simulink model "InjCrv_MI1Cor"  (R2016b)
settings: configuration reference "CodeGenConfigSet" (kept outside this file)
values from neighbouring files (symbols this model uses):
  InjCrv_facMI1APSSOECor_CUR = Calibration.Parameter    [init_InjCrv_MI1Cor.m]
  InjCrv_facMI1APSSOECor_CURX = Calibration.Parameter    [init_InjCrv_MI1Cor.m]
  InjCrv_facMI1ATSSOECor_CUR = Calibration.Parameter    [init_InjCrv_MI1Cor.m]
  InjCrv_facMI1ATSSOECor_CURX = Calibration.Parameter    [init_InjCrv_MI1Cor.m]
  InjCrv_facMI1ETSSOECor_CUR = Calibration.Parameter    [init_InjCrv_MI1Cor.m]
  InjCrv_facMI1ETSSOECor_CURX = Calibration.Parameter    [init_InjCrv_MI1Cor.m]
  InjCrv_phiMI1APSCor1EOM_MAP = Calibration.Parameter    [init_InjCrv_MI1Cor.m]
  InjCrv_phiMI1APSCor1EOM_MAPX = Calibration.Parameter    [init_InjCrv_MI1Cor.m]
  InjCrv_phiMI1APSCor1EOM_MAPY = Calibration.Parameter    [init_InjCrv_MI1Cor.m]
  InjCrv_phiMI1ATSCor1EOM_MAP = Calibration.Parameter    [init_InjCrv_MI1Cor.m]
  InjCrv_phiMI1ATSCor1EOM_MAPX = Calibration.Parameter    [init_InjCrv_MI1Cor.m]
  InjCrv_phiMI1ATSCor1EOM_MAPY = Calibration.Parameter    [init_InjCrv_MI1Cor.m]
  InjCrv_phiMI1ETSCor1EOM_MAP = Calibration.Parameter    [init_InjCrv_MI1Cor.m]
  InjCrv_phiMI1ETSCor1EOM_MAPX = Calibration.Parameter    [init_InjCrv_MI1Cor.m]
  InjCrv_phiMI1ETSCor1EOM_MAPY = Calibration.Parameter    [init_InjCrv_MI1Cor.m]
settings Model: Creator=Administrator  LastModifiedBy=wangrui
settings ConfigSetRef: SourceLocation=Base Workspace

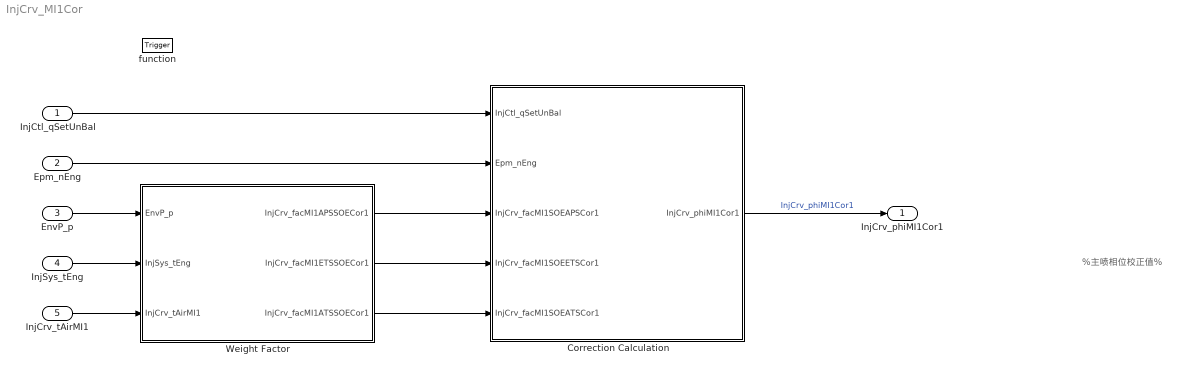
== system InjCrv_MI1Cor ==
  note: %主喷相位校正值%
  InjCtl_qSetUnBal : Inport  Tag=mg/hub  Description=Current injection quantity  OutMin=-319  OutMax=319  OutDataTypeStr=FuelMass_mg_hub
  Epm_nEng : Inport  Tag=rpm  Description=Engine speed  Port=2  OutMin=0  OutMax=6000  OutDataTypeStr=EngSpeed_rpm
  EnvP_p : Inport  Tag=kPa  Description=Barometric pressure  Port=3  OutMin=0  OutMax=3276  OutDataTypeStr=AirPressure_kPa
  InjSys_tEng : Inport  Tag=deg  Description=Engine temperature selected for the injection system  Port=4  OutMin=-1000  OutMax=1000  OutDataTypeStr=Temp_deg
  InjCrv_tAirMI1 : Inport  Tag=deg  Description=Chosen temperature from the temperature field on the induction system  Port=5  OutMin=-50  OutMax=150  OutDataTypeStr=Temp_deg
  function : TriggerPort  TriggerType=function-call  VariantControl=Variant
  Correction Calculation : Subsystem
  Weight Factor : Subsystem
  InjCrv_phiMI1Cor1 : Outport  Tag=CA  Description=Start of energizing correction for MI1  OutMin=-40  OutMax=40  OutDataTypeStr=Angle_CA
  wires:
  EnvP_p/1 -> Weight Factor/1(EnvP_p)
  InjSys_tEng/1 -> Weight Factor/2(InjSys_tEng)
  InjCrv_tAirMI1/1 -> Weight Factor/3(InjCrv_tAirMI1)
  InjCtl_qSetUnBal/1 -> Correction Calculation/1(InjCtl_qSetUnBal)
  Epm_nEng/1 -> Correction Calculation/2(Epm_nEng)
  Weight Factor/1(InjCrv_facMI1APSSOECor1) -> Correction Calculation/3(InjCrv_facMI1SOEAPSCor1)
  Weight Factor/2(InjCrv_facMI1ETSSOECor1) -> Correction Calculation/4(InjCrv_facMI1SOEETSCor1)
  Weight Factor/3(InjCrv_facMI1ATSSOECor1) -> Correction Calculation/5(InjCrv_facMI1SOEATSCor1)
  Correction Calculation/1(InjCrv_phiMI1Cor1) -> InjCrv_phiMI1Cor1/1  "InjCrv_phiMI1Cor1"

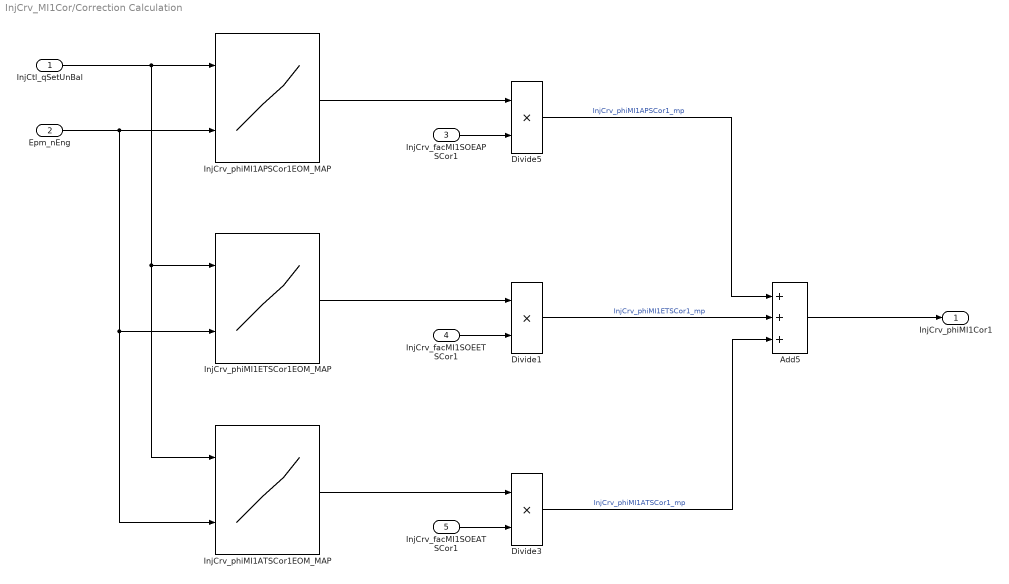
== system InjCrv_MI1Cor/Correction Calculation ==
  InjCtl_qSetUnBal : Inport
  Epm_nEng : Inport  Port=2
  InjCrv_facMI1SOEAPSCor1 : Inport  Port=3
  InjCrv_facMI1SOEETSCor1 : Inport  Port=4
  InjCrv_facMI1SOEATSCor1 : Inport  Port=5
  Add5 : Sum  Inputs=+++  SaturateOnIntegerOverflow=on  InputSameDT=on
  Divide1 : Product  Inputs=**  OutDataTypeStr=Inherit: Inherit via back propagation
  Divide3 : Product  Inputs=**  OutDataTypeStr=Inherit: Inherit via back propagation
  Divide5 : Product  Inputs=**  OutDataTypeStr=Inherit: Inherit via back propagation
  InjCrv_phiMI1APSCor1EOM_MAP : Lookup_n-D  BreakpointsForDimension1=InjCrv_phiMI1APSCor1EOM_MAPY  BreakpointsForDimension2=InjCrv_phiMI1APSCor1EOM_MAPX  IndexSearchMethod=Linear search  BeginIndexSearchUsingPreviousIndexResult=on  Table=InjCrv_phiMI1APSCor1EOM_MAP  ExtrapMethod=Clip  UseLastTableValue=on  InternalRulePriority=Speed  OutDataTypeStr=Inherit: Inherit via back propagation  SaturateOnIntegerOverflow=on
  InjCrv_phiMI1ATSCor1EOM_MAP : Lookup_n-D  BreakpointsForDimension1=InjCrv_phiMI1ATSCor1EOM_MAPY  BreakpointsForDimension2=InjCrv_phiMI1ATSCor1EOM_MAPX  IndexSearchMethod=Linear search  BeginIndexSearchUsingPreviousIndexResult=on  Table=InjCrv_phiMI1ATSCor1EOM_MAP  ExtrapMethod=Clip  UseLastTableValue=on  InternalRulePriority=Speed  OutDataTypeStr=Inherit: Inherit via back propagation  SaturateOnIntegerOverflow=on
  InjCrv_phiMI1ETSCor1EOM_MAP : Lookup_n-D  BreakpointsForDimension1=InjCrv_phiMI1ETSCor1EOM_MAPY  BreakpointsForDimension2=InjCrv_phiMI1ETSCor1EOM_MAPX  IndexSearchMethod=Linear search  BeginIndexSearchUsingPreviousIndexResult=on  Table=InjCrv_phiMI1ETSCor1EOM_MAP  ExtrapMethod=Clip  UseLastTableValue=on  InternalRulePriority=Speed  OutDataTypeStr=Inherit: Inherit via back propagation  SaturateOnIntegerOverflow=on
  InjCrv_phiMI1Cor1 : Outport
  wires:
  InjCrv_phiMI1APSCor1EOM_MAP/1 -> Divide5/1
  InjCrv_facMI1SOEAPSCor1/1 -> Divide5/2
  Divide5/1 -> Add5/1  "InjCrv_phiMI1APSCor1_mp"
  InjCrv_phiMI1ETSCor1EOM_MAP/1 -> Divide1/1
  InjCrv_facMI1SOEETSCor1/1 -> Divide1/2
  InjCrv_phiMI1ATSCor1EOM_MAP/1 -> Divide3/1
  InjCrv_facMI1SOEATSCor1/1 -> Divide3/2
  Divide3/1 -> Add5/3  "InjCrv_phiMI1ATSCor1_mp"
  Add5/1 -> InjCrv_phiMI1Cor1/1
  Divide1/1 -> Add5/2  "InjCrv_phiMI1ETSCor1_mp"
  InjCtl_qSetUnBal/1 -> InjCrv_phiMI1ATSCor1EOM_MAP/1, InjCrv_phiMI1ETSCor1EOM_MAP/1, InjCrv_phiMI1APSCor1EOM_MAP/1
  Epm_nEng/1 -> InjCrv_phiMI1ATSCor1EOM_MAP/2, InjCrv_phiMI1ETSCor1EOM_MAP/2, InjCrv_phiMI1APSCor1EOM_MAP/2

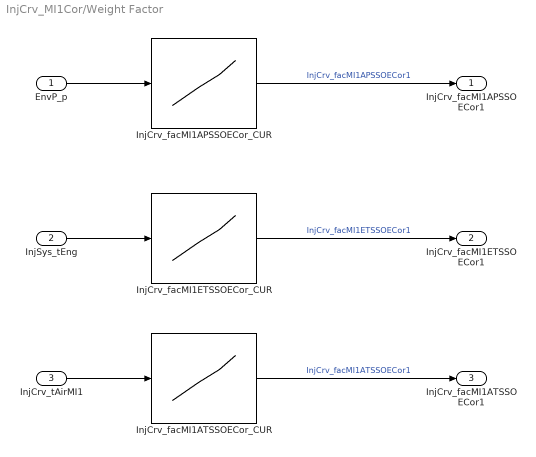
== system InjCrv_MI1Cor/Weight Factor ==
  EnvP_p : Inport
  InjSys_tEng : Inport  Port=2
  InjCrv_tAirMI1 : Inport  Port=3
  InjCrv_facMI1APSSOECor_CUR : Lookup_n-D  NumberOfTableDimensions=1  BreakpointsForDimension1=InjCrv_facMI1APSSOECor_CURX  IndexSearchMethod=Linear search  BeginIndexSearchUsingPreviousIndexResult=on  Table=InjCrv_facMI1APSSOECor_CUR  ExtrapMethod=Clip  UseLastTableValue=on  InternalRulePriority=Speed  OutDataTypeStr=Inherit: Inherit via back propagation  SaturateOnIntegerOverflow=on
  InjCrv_facMI1ATSSOECor_CUR : Lookup_n-D  NumberOfTableDimensions=1  BreakpointsForDimension1=InjCrv_facMI1ATSSOECor_CURX  IndexSearchMethod=Linear search  BeginIndexSearchUsingPreviousIndexResult=on  Table=InjCrv_facMI1ATSSOECor_CUR  ExtrapMethod=Clip  UseLastTableValue=on  InternalRulePriority=Speed  OutDataTypeStr=Inherit: Inherit via back propagation  SaturateOnIntegerOverflow=on
  InjCrv_facMI1ETSSOECor_CUR : Lookup_n-D  NumberOfTableDimensions=1  BreakpointsForDimension1=InjCrv_facMI1ETSSOECor_CURX  IndexSearchMethod=Linear search  BeginIndexSearchUsingPreviousIndexResult=on  Table=InjCrv_facMI1ETSSOECor_CUR  ExtrapMethod=Clip  UseLastTableValue=on  InternalRulePriority=Speed  OutDataTypeStr=Inherit: Inherit via back propagation  SaturateOnIntegerOverflow=on
  InjCrv_facMI1APSSOECor1 : Outport
  InjCrv_facMI1ETSSOECor1 : Outport  Port=2
  InjCrv_facMI1ATSSOECor1 : Outport  Port=3
  wires:
  InjCrv_facMI1APSSOECor_CUR/1 -> InjCrv_facMI1APSSOECor1/1  "InjCrv_facMI1APSSOECor1"
  InjCrv_facMI1ETSSOECor_CUR/1 -> InjCrv_facMI1ETSSOECor1/1  "InjCrv_facMI1ETSSOECor1"
  InjCrv_facMI1ATSSOECor_CUR/1 -> InjCrv_facMI1ATSSOECor1/1  "InjCrv_facMI1ATSSOECor1"
  EnvP_p/1 -> InjCrv_facMI1APSSOECor_CUR/1
  InjSys_tEng/1 -> InjCrv_facMI1ETSSOECor_CUR/1
  InjCrv_tAirMI1/1 -> InjCrv_facMI1ATSSOECor_CUR/1
